simulink model "PVTOL_PseudoSMC"  (R2026b)
settings Model: Creator=nestorhernandezcastellanos  LastModifiedBy=nestorhernandezcastellanos

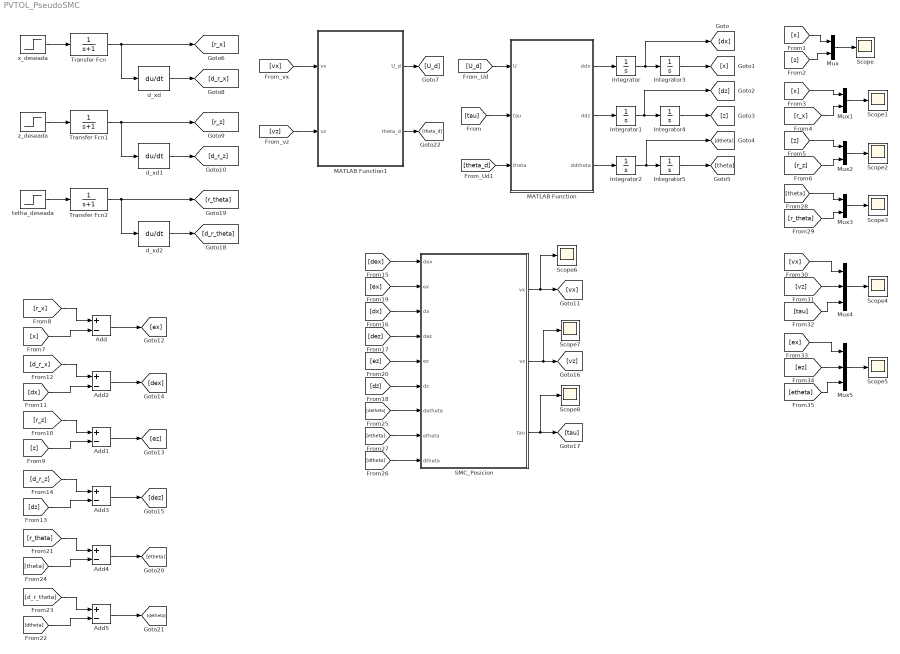
== system PVTOL_PseudoSMC ==
  Add{,1..5} (6 alike) : Sum  Inputs=+-
  Integrator : Integrator  InitialCondition=2
  Integrator1 : Integrator  InitialCondition=3
  Integrator2 : Integrator  InitialCondition=15
  Integrator3 : Integrator  InitialCondition=2
  Integrator4 : Integrator  InitialCondition=3
  Integrator5 : Integrator  InitialCondition=15
  MATLAB Function : MATLAB Function  TreatAsAtomicUnit=on
  MATLAB Function1 : MATLAB Function  TreatAsAtomicUnit=on
  Mux{,1..3} (4 alike) : Mux  Inputs=2
  Mux4 : Mux  Inputs=3
  Mux5 : Mux  Inputs=3
  SMC_Posicion : MATLAB Function  TreatAsAtomicUnit=on
  Scope{,1..8} (9 alike) : Scope
      Scope settings: ActiveDisplayYMinimum=0.024738728132078558  ActiveDisplayYMaximum=5.5528067767038412
      Scope1 settings: ActiveDisplayYMinimum=-0.62499999649831228  ActiveDisplayYMaximum=5.6249999684848113
      Scope2 settings: ActiveDisplayYMinimum=-0.62499999649831228  ActiveDisplayYMaximum=5.6249999684848113  DataLoggingVariableName=ScopeData2
      Scope3 settings: ActiveDisplayYMinimum=-2.37928301075874  ActiveDisplayYMaximum=21.413547096828665  DataLoggingVariableName=ScopeData3
      Scope4 settings: ActiveDisplayYMinimum=-47.002794390550264  ActiveDisplayYMaximum=23.025149514952403  DataLoggingVariableName=ScopeData4
      Scope5 settings: ActiveDisplayYMinimum=-21.515656728928203  ActiveDisplayYMaximum=3.2982696996545835  DataLoggingVariableName=ScopeData5
      Scope6 settings: ActiveDisplayYMinimum=-21.515643312433614  ActiveDisplayYMaximum=3.2981489512032809  DataLoggingVariableName=ScopeData6
      Scope7 settings: ActiveDisplayYMinimum=-21.515643312433614  ActiveDisplayYMaximum=3.2981489512032809  DataLoggingVariableName=ScopeData7
      Scope8 settings: ActiveDisplayYMinimum=-21.515643312433614  ActiveDisplayYMaximum=3.2981489512032809  DataLoggingVariableName=ScopeData8
  Transfer Fcn : TransferFcn  Denominator=[1 1]
  Transfer Fcn1 : TransferFcn  Denominator=[1 1]
  Transfer Fcn2 : TransferFcn  Denominator=[1 1]
  d_xd : Derivative
  d_xd1 : Derivative
  d_xd2 : Derivative
  tetha_deseada : Step  FinalValue=5  SampleTime=0
  x_deseada : Step  FinalValue=5  SampleTime=0
  z_deseada : Step  FinalValue=5  SampleTime=0
  wires:
  MATLAB Function/1(ddx) -> Integrator/1
  MATLAB Function/2(ddz) -> Integrator1/1
  MATLAB Function/3(ddtheta) -> Integrator2/1
  Integrator2/1 -> [dtheta], Integrator5/1
  Integrator1/1 -> [dz], Integrator4/1
  Integrator/1 -> [dx], Integrator3/1
  Integrator3/1 -> [x]
  Integrator4/1 -> [z]
  Integrator5/1 -> [theta]
  Mux/1 -> Scope/1
  [z] -> Mux/2
  [x] -> Mux/1
  x_deseada/1 -> Transfer Fcn/1
  Transfer Fcn/1 -> [r_x], d_xd/1
  [vx] -> MATLAB Function1/1(vx)
  [vz] -> MATLAB Function1/2(vz)
  [U_d] -> MATLAB Function/1(U)
  MATLAB Function1/1(U_d) -> [U_d]
  [x] -> Mux1/1
  [r_x] -> Mux1/2
  Mux1/1 -> Scope1/1
  Mux2/1 -> Scope2/1
  [r_z] -> Mux2/2
  [z] -> Mux2/1
  d_xd/1 -> [d_r_x]
  d_xd1/1 -> [d_r_z]
  Transfer Fcn1/1 -> d_xd1/1, [r_z]
  z_deseada/1 -> Transfer Fcn1/1
  [tau] -> MATLAB Function/2(tau)
  [r_x] -> Add/1
  [x] -> Add/2
  Add/1 -> [ex]
  Add1/1 -> [ez]
  [z] -> Add1/2
  [r_z] -> Add1/1
  Add2/1 -> [dex]
  [dx] -> Add2/2
  [d_r_x] -> Add2/1
  [d_r_z] -> Add3/1
  [dz] -> Add3/2
  Add3/1 -> [dez]
  SMC_Posicion/1(vx) -> Scope6/1, [vx]
  SMC_Posicion/2(vz) -> Scope7/1, [vz]
  SMC_Posicion/3(tau) -> Scope8/1, [tau]
  [dex] -> SMC_Posicion/1(dex)
  [dx] -> SMC_Posicion/3(dx)
  [dez] -> SMC_Posicion/4(dez)
  [dz] -> SMC_Posicion/6(dz)
  [ex] -> SMC_Posicion/2(ex)
  [ez] -> SMC_Posicion/5(ez)
  tetha_deseada/1 -> Transfer Fcn2/1
  Transfer Fcn2/1 -> [r_theta], d_xd2/1
  d_xd2/1 -> [d_r_theta]
  Add5/1 -> [detheta]
  [dtheta] -> Add5/2
  [d_r_theta] -> Add5/1
  [r_theta] -> Add4/1
  [theta] -> Add4/2
  Add4/1 -> [etheta]
  [detheta] -> SMC_Posicion/7(detheta)
  [etheta] -> SMC_Posicion/8(etheta)
  [dtheta] -> SMC_Posicion/9(dtheta)
  MATLAB Function1/2(theta_d) -> [theta_d]
  [theta_d] -> MATLAB Function/3(theta)
  [theta] -> Mux3/1
  [r_theta] -> Mux3/2
  Mux3/1 -> Scope3/1
  Mux4/1 -> Scope4/1
  [vz] -> Mux4/2
  [vx] -> Mux4/1
  [tau] -> Mux4/3
  [etheta] -> Mux5/3
  [ex] -> Mux5/1
  [ez] -> Mux5/2
  Mux5/1 -> Scope5/1

== matlab function PVTOL_PseudoSMC/MATLAB Function1 ==
  data: vx input; U_d output; vz input; theta_d output
function [U_d,theta_d] = linealizacion(vx,vz)

g = 9.81;                                  
U_d = sqrt(vx^2 + (vz+g)^2);                 
theta_d = atan2(-vx,vz+g);

== matlab function PVTOL_PseudoSMC/MATLAB Function ==
  data: U input; ddx output; tau input; theta input; ddz output; ddtheta output
function [ddx,ddz,ddtheta] = planta(U,tau,theta)

g = 9.81;                                       

ddx = -U*sin(theta);                            
ddz = U*cos(theta)-g;                           
ddtheta = tau;

== matlab function PVTOL_PseudoSMC/SMC_Posicion ==
  data: dex input; ex input; dx input; vx output; dez input; ez input; dz input; vz output; tau output; detheta input; etheta input; dtheta input
function [vx, vz, tau] = controlador(dex, ex, dx, dez, ez, dz, detheta, etheta, dtheta)

% Parámetros de las superficies de deslizamiento
mx = 2;
mz = 2;
mtheta = 2;

% Ganancias del controlador
Kx = 10;
Kz = 10;
Ktheta = 10;

% Amplitudes de las funciones de saturación
Lx = 1;
Lz = 1;
Ltheta = 1;

% Parámetros de pendiente
eta_x = 0.05;
eta_z = 0.05;
eta_theta = 0.05;

% Superficies de pseudo modo deslizante
sigma_x = dex + mx*ex;
sigma_z = dez + mz*ez;
sigma_theta = detheta + mtheta*etheta;

% Funciones de saturación
sat_x = max(-Lx, min(Lx, sigma_x/eta_x));
sat_z = max(-Lz, min(Lz, sigma_z/eta_z));
sat_theta = max(-Ltheta, min(Ltheta, sigma_theta/eta_theta));

% Entradas virtuales
vx = -mx*dx + Kx*sat_x;
vz = -mz*dz + Kz*sat_z;

% Control de actitud
tau = -mtheta*dtheta + Ktheta*sat_theta;
